simulink model "maglev_2d"  (R2022b)
settings: Solver=VariableStepAuto  StartTime=0.0  StopTime=1  RelTol=1e-3
model workspace (MAT data in the model file):
  params.solenoids.x = [0.02 -0.02 0 0]
  params.solenoids.y = [0 0 0.02 -0.02]
  params.solenoids.r = [0.00925 0.00925 0.00925 0.00925]
  params.solenoids.l = [0.012 0.012 0.012 0.012]
  params.solenoids.z = [0.006 0.006 0.006 0.006]
  params.solenoids.nw = 480
  params.permanent.x = [0.028 -0.028 0.028 -0.028]
  params.permanent.y = [0.028 0.028 -0.028 -0.028]
  params.permanent.r = [0.01 0.01 0.01 0.01]
  params.permanent.l = [0.009 0.009 0.009 0.009]
  params.permanent.z = [0.0046 0.0046 0.0046 0.0046]
  params.permanent.J = 1.1
  params.magnet.r = 0.025
  params.magnet.l = 0.005
  params.magnet.J = -1
  params.magnet.m = 0.077
  params.magnet.I = [1.21916666667e-05 1.21916666667e-05 2.40625e-05]
  params.magnet.n = 100
  params.sensors.x = [0 -0.019 -0.019]
  params.sensors.y = [0 0.019 -0.019]
  params.sensors.z = [0 0 0]
  params.physical.g = 9.81
  params.physical.mu0 = 1.25663706144e-06
settings Model: ParameterArgumentNames=params  Creator=hansae  LastModifiedBy=hansae

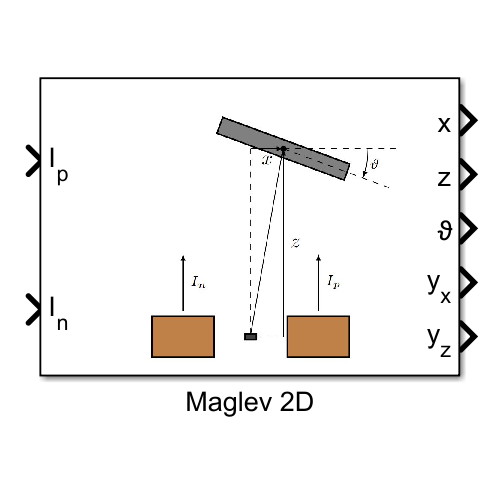
[thumbnail: Simulink's stored preview of the top-level diagram]
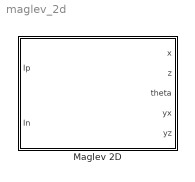
== system maglev_2d ==
  Maglev 2D : Subsystem
      mask Display:
      | image('$imagefile'); % Use "Edit Image" on toolstrip to change.
      | port_label('input', 1, 'I_p','interpreter','tex')
      | port_label('input', 2, 'I_n','interpreter','tex')
      | port_label('output', 1, 'x','interpreter','tex')
      | port_label('output', 2, 'z','interpreter','tex')
      | port_label('output', 3, '\vartheta','interpreter','tex')
      | port_label('output', 4, 'y_x','interpreter','tex')
      | port_label('output', 5, 'y_z','interpreter','tex')

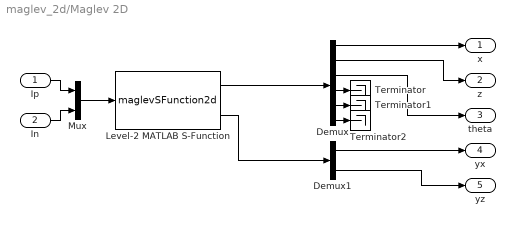
== system maglev_2d/Maglev 2D ==
  Ip : Inport
  In : Inport  Port=2
  Demux : Demux  Outputs=6
  Demux1 : Demux  Outputs=2
  Level-2 MATLAB S-Function : M-S-Function  FunctionName=maglevSFunction2d
  Mux : Mux  Inputs=2
  Terminator : Terminator
  Terminator1 : Terminator
  Terminator2 : Terminator
  x : Outport
  z : Outport  Port=2
  theta : Outport  Port=3
  yx : Outport  Port=4
  yz : Outport  Port=5
  wires:
  Demux/1 -> x/1
  Demux/3 -> theta/1
  Demux1/1 -> yx/1
  Demux1/2 -> yz/1
  Mux/1 -> Level-2 MATLAB S-Function/1
  Ip/1 -> Mux/1
  In/1 -> Mux/2
  Demux/4 -> Terminator/1
  Demux/5 -> Terminator1/1
  Demux/6 -> Terminator2/1
  Level-2 MATLAB S-Function/2 -> Demux1/1
  Level-2 MATLAB S-Function/1 -> Demux/1
  Demux/2 -> z/1
